simulink model "satellite_GVE_per_model_formation_sim"  (R2021a)
settings: Solver=VariableStepAuto  StartTime=0  StopTime=10800  FixedStep=1  RelTol=1e-3
values from neighbouring files (symbols this model uses):
  a_ini = (960e3+1019e3)/2+R_e    (= 7367700)    [Satellite_MPC3.m]
  Cd = 2.2    [Satellite_MPC3.m]
  e_ini = 0.0039866    [Satellite_MPC3.m]
  Form_dis = 1e3    (= 1000)    [Satellite_MPC3.m]
  i_ini = 82.9236/180*pi()    [Satellite_MPC3.m]
  J2 = 1082.63e-6    (= 0.00108263)    [Satellite_MPC3.m]
  K = 2    [Satellite_MPC3.m]
  kd = 0    [Satellite_MPC3.m]
  ki = 0    [Satellite_MPC3.m]
  kp = 4e-7    (= 4e-07)    [Satellite_MPC3.m]
  m_s = 27    [Satellite_MPC3.m]
  meu = G*m_e    (= 397865500000000)    [Satellite_MPC3.m]
  Ohm_ini = 272.9481/180*pi()    [Satellite_MPC3.m]
  p_solar = 4.65e-06    [Satellite_MPC3.m]
  R_e = 6378.2e3    (= 6378200)    [Satellite_MPC3.m]
  s = 0.2*0.2    (= 0.04)    [Satellite_MPC3.m]
  theta1_ini = 0    [Satellite_MPC3.m]
  theta2_ini = 1e-7    (= 1e-07)    [Satellite_MPC3.m]
  theta3_ini = 2e-7    (= 2e-07)    [Satellite_MPC3.m]
  theta_ini = 0    [Satellite_MPC3.m]
  u_lim = inf    [Satellite_MPC3.m]
  w_ini = 297.2910/180*pi()    [Satellite_MPC3.m]
libraries: pid_lib x3
(part 2 of 2)

== system satellite_GVE_per_model_formation_sim/RTN2ECI_SatPer_Sys1/RTN2OE_SatPer_Sys/atm_darg_acc/Pressure of r ==
  T : Inport
  Constant : Constant  Value=2.448
  Constant5 : Constant  Value=273.1
  Constant7 : Constant  Value=216.6
  Constant8 : Constant  Value=11.388
  Math Function : Math  Operator=pow  SaturateOnIntegerOverflow=on
  Product : Product  Inputs=*/
  Product23 : Product  Inputs=*/
  Sum8 : Sum  Inputs=|++
  p : Outport
  wires:
  Constant/1 -> Product/1
  Math Function/1 -> Product/2
  Product23/1 -> Math Function/2
  Constant7/1 -> Product23/2
  Sum8/1 -> Product23/1
  Constant8/1 -> Math Function/1
  T/1 -> Sum8/1
  Product/1 -> p/1  "p"
  Constant5/1 -> Sum8/2

== system satellite_GVE_per_model_formation_sim/RTN2ECI_SatPer_Sys1/RTN2OE_SatPer_Sys/atm_darg_acc/Tem of r ==
  In1 : Inport
  Constant5 : Constant  Value=-131.21
  Gain : Gain  Gain=0.00299
  Sum8 : Sum  Inputs=|++
  T : Outport
  wires:
  In1/1 -> Gain/1
  Constant5/1 -> Sum8/2
  Gain/1 -> Sum8/1
  Sum8/1 -> T/1  "T"

== system satellite_GVE_per_model_formation_sim/RTN2ECI_SatPer_Sys1/RTN2OE_SatPer_Sys/atm_darg_acc/atm_dens of r ==
  p : Inport
  T : Inport  Port=2
  Constant5 : Constant  Value=0.2869
  Constant7 : Constant  Value=273.1
  Product23 : Product  Inputs=*//
  Sum8 : Sum  Inputs=|++
  atm_dens : Outport
  wires:
  p/1 -> Product23/1
  Product23/1 -> atm_dens/1  "atm_dens"
  Constant7/1 -> Sum8/2
  Sum8/1 -> Product23/2
  Constant5/1 -> Product23/3
  T/1 -> Sum8/1

== system satellite_GVE_per_model_formation_sim/RTN2ECI_SatPer_Sys2/RTN2OE_SatPer_Sys/atm_darg_acc/Pressure of r ==
  T : Inport
  Constant : Constant  Value=2.448
  Constant5 : Constant  Value=273.1
  Constant7 : Constant  Value=216.6
  Constant8 : Constant  Value=11.388
  Math Function : Math  Operator=pow  SaturateOnIntegerOverflow=on
  Product : Product  Inputs=*/
  Product23 : Product  Inputs=*/
  Sum8 : Sum  Inputs=|++
  p : Outport
  wires:
  Constant5/1 -> Sum8/2
  Product/1 -> p/1  "p"
  T/1 -> Sum8/1
  Constant8/1 -> Math Function/1
  Sum8/1 -> Product23/1
  Constant7/1 -> Product23/2
  Product23/1 -> Math Function/2
  Math Function/1 -> Product/2
  Constant/1 -> Product/1

== system satellite_GVE_per_model_formation_sim/RTN2ECI_SatPer_Sys2/RTN2OE_SatPer_Sys/atm_darg_acc/Tem of r ==
  In1 : Inport
  Constant5 : Constant  Value=-131.21
  Gain : Gain  Gain=0.00299
  Sum8 : Sum  Inputs=|++
  T : Outport
  wires:
  Sum8/1 -> T/1  "T"
  Gain/1 -> Sum8/1
  Constant5/1 -> Sum8/2
  In1/1 -> Gain/1

== system satellite_GVE_per_model_formation_sim/RTN2ECI_SatPer_Sys2/RTN2OE_SatPer_Sys/atm_darg_acc/atm_dens of r ==
  p : Inport
  T : Inport  Port=2
  Constant5 : Constant  Value=0.2869
  Constant7 : Constant  Value=273.1
  Product23 : Product  Inputs=*//
  Sum8 : Sum  Inputs=|++
  atm_dens : Outport
  wires:
  T/1 -> Sum8/1
  Constant5/1 -> Product23/3
  Sum8/1 -> Product23/2
  Constant7/1 -> Sum8/2
  Product23/1 -> atm_dens/1  "atm_dens"
  p/1 -> Product23/1

== matlab function satellite_GVE_per_model_formation_sim/ECI2RTN ==
  data: u_I input; u_rtn output; w input; theta input; Ohm input; inc input
function u_rtn  = fcn(u_I,w,theta,Ohm,inc)
u = w+theta;
C_oI = [-sin(u)*cos(Ohm)-cos(u)*cos(inc)*sin(Ohm) -sin(u)*sin(Ohm)+cos(u)*cos(inc)*cos(Ohm) cos(u)*sin(inc);
            -sin(inc)*sin(Ohm)                        sin(inc)*cos(Ohm)                         -cos(inc);
            -cos(u)*cos(Ohm)+sin(u)*cos(inc)*sin(Ohm) -cos(u)*sin(Ohm)-sin(u)*cos(inc)*cos(Ohm) -sin(u)*sin(inc)];
C_rtno = [0 0 -1;1 0 0;0 -1 0];
u_rtn = C_rtno*C_oI*u_I;

== matlab function satellite_GVE_per_model_formation_sim/ECI2OE ==
  data: pos input; a output; vel input; meu input; e output; i output; w output; Ohm output; theta output
function [a,e,i,w,Ohm,theta] = fcn(pos,vel,meu)
x_v = [1;0;0];
z_v = [0;0;1];    
y_v = [0;1;0];
a = (2/norm(pos)-norm(vel)^2/meu)^-1;
e_v = [(norm(vel)^2-meu/norm(pos))*pos-dot(pos,vel)*vel]/meu;
e = norm(e_v);
h_v = cross(pos,vel);
i = acos(dot(z_v,h_v)/norm(h_v));
n_v = cross(z_v,h_v);
if dot(z_v,e_v)>0
   w = acos(dot(n_v,e_v)/norm(n_v)/e);
else
   w = pi()+acos(dot(n_v,e_v)/norm(n_v)/e);
end
if dot(y_v,n_v)>0
    Ohm = acos(dot(n_v,x_v)/norm(n_v));
else
    Ohm = pi()+ acos(dot(n_v,x_v)/norm(n_v));
end
if dot(pos,vel)>0
    theta = acos(dot(e_v,pos)/e/norm(pos));
else
    theta = pi()+acos(dot(e_v,pos)/e/norm(pos));
end

== matlab function satellite_GVE_per_model_formation_sim/OE&ECI_RefOrbit/velosity vector ==
  data: meu input; p input; Ohm input; y output; w input; theta input; i input; e input
function y = fcn(meu,p,Ohm,w,theta,i,e)
    vel_vec = sqrt(meu/p)*[-cos(Ohm)*(sin(w+theta)+e*sin(w))-sin(Ohm)*(cos(w+theta)+e*cos(w))*cos(i);
                           -sin(Ohm)*(sin(w+theta)+e*sin(w))+cos(Ohm)*(cos(w+theta)+e*cos(w))*cos(i);
                           (cos(w+theta)+e*cos(w))*sin(i)];
y = vel_vec;

== matlab function satellite_GVE_per_model_formation_sim/RTN2ECI_SatPer_Sys/RTN2OE_SatPer_Sys/velosity vector ==
  data: meu input; p input; Ohm input; y output; w input; theta input; i input; e input
function y = fcn(meu,p,Ohm,w,theta,i,e)
    vel_vec = sqrt(meu/p)*[-cos(Ohm)*(sin(w+theta)+e*sin(w))-sin(Ohm)*(cos(w+theta)+e*cos(w))*cos(i);
                           -sin(Ohm)*(sin(w+theta)+e*sin(w))+cos(Ohm)*(cos(w+theta)+e*cos(w))*cos(i);
                           (cos(w+theta)+e*cos(w))*sin(i)];
y = vel_vec;

== matlab function satellite_GVE_per_model_formation_sim/RTN2ECI_SatPer_Sys1/RTN2OE_SatPer_Sys/velosity vector ==
  data: meu input; p input; Ohm input; y output; w input; theta input; i input; e input
function y = fcn(meu,p,Ohm,w,theta,i,e)
    vel_vec = sqrt(meu/p)*[-cos(Ohm)*(sin(w+theta)+e*sin(w))-sin(Ohm)*(cos(w+theta)+e*cos(w))*cos(i);
                           -sin(Ohm)*(sin(w+theta)+e*sin(w))+cos(Ohm)*(cos(w+theta)+e*cos(w))*cos(i);
                           (cos(w+theta)+e*cos(w))*sin(i)];
y = vel_vec;

== matlab function satellite_GVE_per_model_formation_sim/RTN2ECI_SatPer_Sys2/RTN2OE_SatPer_Sys/velosity vector ==
  data: meu input; p input; Ohm input; y output; w input; theta input; i input; e input
function y = fcn(meu,p,Ohm,w,theta,i,e)
    vel_vec = sqrt(meu/p)*[-cos(Ohm)*(sin(w+theta)+e*sin(w))-sin(Ohm)*(cos(w+theta)+e*cos(w))*cos(i);
                           -sin(Ohm)*(sin(w+theta)+e*sin(w))+cos(Ohm)*(cos(w+theta)+e*cos(w))*cos(i);
                           (cos(w+theta)+e*cos(w))*sin(i)];
y = vel_vec;

== matlab function satellite_GVE_per_model_formation_sim/ECI2RTN1 ==
  data: u_I input; u_rtn output; w input; theta input; Ohm input; inc input
function u_rtn  = fcn(u_I,w,theta,Ohm,inc)
u = w+theta;
C_oI = [-sin(u)*cos(Ohm)-cos(u)*cos(inc)*sin(Ohm) -sin(u)*sin(Ohm)+cos(u)*cos(inc)*cos(Ohm) cos(u)*sin(inc);
            -sin(inc)*sin(Ohm)                        sin(inc)*cos(Ohm)                         -cos(inc);
            -cos(u)*cos(Ohm)+sin(u)*cos(inc)*sin(Ohm) -cos(u)*sin(Ohm)-sin(u)*cos(inc)*cos(Ohm) -sin(u)*sin(inc)];
C_rtno = [0 0 -1;1 0 0;0 -1 0];
u_rtn = C_rtno*C_oI*u_I;

== matlab function satellite_GVE_per_model_formation_sim/RTN2ECI_SatPer_Sys/Position unit vector ==
  data: Ohm input; y output; w input; theta input; i input
function y = fcn(Ohm,w,theta,i)
    unit_vec = [cos(Ohm)*cos(w+theta)-sin(Ohm)*sin(w+theta)*cos(i);
                sin(Ohm)*cos(w+theta)+cos(Ohm)*sin(w+theta)*cos(i);
                sin(w+theta)*sin(i)];
y = unit_vec;

== matlab function satellite_GVE_per_model_formation_sim/ECI2RTN2 ==
  data: u_I input; u_rtn output; w input; theta input; Ohm input; inc input
function u_rtn  = fcn(u_I,w,theta,Ohm,inc)
u = w+theta;
C_oI = [-sin(u)*cos(Ohm)-cos(u)*cos(inc)*sin(Ohm) -sin(u)*sin(Ohm)+cos(u)*cos(inc)*cos(Ohm) cos(u)*sin(inc);
            -sin(inc)*sin(Ohm)                        sin(inc)*cos(Ohm)                         -cos(inc);
            -cos(u)*cos(Ohm)+sin(u)*cos(inc)*sin(Ohm) -cos(u)*sin(Ohm)-sin(u)*cos(inc)*cos(Ohm) -sin(u)*sin(inc)];
C_rtno = [0 0 -1;1 0 0;0 -1 0];
u_rtn = C_rtno*C_oI*u_I;

== matlab function satellite_GVE_per_model_formation_sim/RTN2ECI_SatPer_Sys/RTN2OE_SatPer_Sys/Solar Pressure Acc Compute ==
  data: K_all input; w input; y output; theta input; Ohm input; inc input; SE_vector input
function y = fcn(K_all,w,theta,Ohm,inc,SE_vector)
if((theta>168*pi()/180)&&(theta<278*pi()/180))
    C_oI = zeros(3,3);
    C_rtno = zeros(3,3);
else
    u = w+theta;
    C_oI = [-sin(u)*cos(Ohm)-cos(u)*cos(inc)*sin(Ohm) -sin(u)*sin(Ohm)+cos(u)*cos(inc)*cos(Ohm) cos(u)*sin(inc);
            -sin(inc)*sin(Ohm)                        sin(inc)*cos(Ohm)                         -cos(inc);
            -cos(u)*cos(Ohm)+sin(u)*cos(inc)*sin(Ohm) -cos(u)*sin(Ohm)-sin(u)*cos(inc)*cos(Ohm) -sin(u)*sin(inc)];
    C_rtno = [0 0 -1;1 0 0;0 -1 0];
end
y = K_all*C_rtno*C_oI*SE_vector;

== matlab function satellite_GVE_per_model_formation_sim/OE&ECI_RefOrbit/Refpos unit vector ==
  data: Ohm input; y output; w input; theta input; i input
function y = fcn(Ohm,w,theta,i)
    unit_vec = [cos(Ohm)*cos(w+theta)-sin(Ohm)*sin(w+theta)*cos(i);
                sin(Ohm)*cos(w+theta)+cos(Ohm)*sin(w+theta)*cos(i);
                sin(w+theta)*sin(i)];
y = unit_vec;

== matlab function satellite_GVE_per_model_formation_sim/RTN2ECI_SatPer_Sys1/RTN2OE_SatPer_Sys/Solar Pressure Acc Compute ==
  data: K_all input; w input; y output; theta input; Ohm input; inc input; SE_vector input
function y = fcn(K_all,w,theta,Ohm,inc,SE_vector)
if((theta>168*pi()/180)&&(theta<278*pi()/180))
    C_oI = zeros(3,3);
    C_rtno = zeros(3,3);
else
    u = w+theta;
    C_oI = [-sin(u)*cos(Ohm)-cos(u)*cos(inc)*sin(Ohm) -sin(u)*sin(Ohm)+cos(u)*cos(inc)*cos(Ohm) cos(u)*sin(inc);
            -sin(inc)*sin(Ohm)                        sin(inc)*cos(Ohm)                         -cos(inc);
            -cos(u)*cos(Ohm)+sin(u)*cos(inc)*sin(Ohm) -cos(u)*sin(Ohm)-sin(u)*cos(inc)*cos(Ohm) -sin(u)*sin(inc)];
    C_rtno = [0 0 -1;1 0 0;0 -1 0];
end
y = K_all*C_rtno*C_oI*SE_vector;

== matlab function satellite_GVE_per_model_formation_sim/RTN2ECI_SatPer_Sys1/Position unit vector ==
  data: Ohm input; y output; w input; theta input; i input
function y = fcn(Ohm,w,theta,i)
    unit_vec = [cos(Ohm)*cos(w+theta)-sin(Ohm)*sin(w+theta)*cos(i);
                sin(Ohm)*cos(w+theta)+cos(Ohm)*sin(w+theta)*cos(i);
                sin(w+theta)*sin(i)];
y = unit_vec;

== matlab function satellite_GVE_per_model_formation_sim/RTN2ECI_SatPer_Sys2/RTN2OE_SatPer_Sys/Solar Pressure Acc Compute ==
  data: K_all input; w input; y output; theta input; Ohm input; inc input; SE_vector input
function y = fcn(K_all,w,theta,Ohm,inc,SE_vector)
if((theta>168*pi()/180)&&(theta<278*pi()/180))
    C_oI = zeros(3,3);
    C_rtno = zeros(3,3);
else
    u = w+theta;
    C_oI = [-sin(u)*cos(Ohm)-cos(u)*cos(inc)*sin(Ohm) -sin(u)*sin(Ohm)+cos(u)*cos(inc)*cos(Ohm) cos(u)*sin(inc);
            -sin(inc)*sin(Ohm)                        sin(inc)*cos(Ohm)                         -cos(inc);
            -cos(u)*cos(Ohm)+sin(u)*cos(inc)*sin(Ohm) -cos(u)*sin(Ohm)-sin(u)*cos(inc)*cos(Ohm) -sin(u)*sin(inc)];
    C_rtno = [0 0 -1;1 0 0;0 -1 0];
end
y = K_all*C_rtno*C_oI*SE_vector;

== matlab function satellite_GVE_per_model_formation_sim/RTN2ECI_SatPer_Sys2/Position unit vector ==
  data: Ohm input; y output; w input; theta input; i input
function y = fcn(Ohm,w,theta,i)
    unit_vec = [cos(Ohm)*cos(w+theta)-sin(Ohm)*sin(w+theta)*cos(i);
                sin(Ohm)*cos(w+theta)+cos(Ohm)*sin(w+theta)*cos(i);
                sin(w+theta)*sin(i)];
y = unit_vec;

== matlab function satellite_GVE_per_model_formation_sim/Formation_com ==
  data: p1 input; v_12 output; p2 input; p3 input; v_13 output; v_23 output; d12 output; d13 output; d23 output
function [v_12,v_13,v_23,d12,d13,d23] = fcn(p1,p2,p3)
d12 = norm(p1-p2);
d13 = norm(p1-p3);
d23 = norm(p2-p3);
v_12 = (p2-p1)/d12;
v_13 = (p3-p1)/d13;
v_23 = (p3-p2)/d23;
